simulink model "quad_waypoint_schedule"  (R2020a)
settings: Solver=FixedStepAuto  StartTime=0.0  StopTime=10.0  RelTol=1e-3
undefined symbols (not defined in the file): sim_freq, threshold, waypoints, waypoints_time
libraries: simulink x1
settings Model: Creator=francois  LastModifiedBy=murray

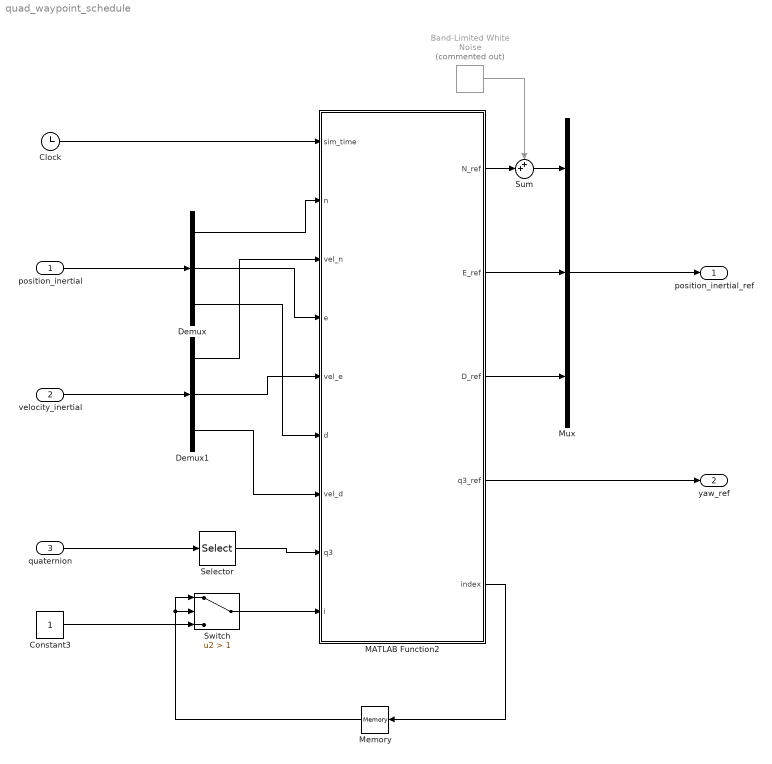
== system quad_waypoint_schedule ==
  position_inertial : Inport
  velocity_inertial : Inport  Port=2
  quaternion : Inport  Port=3
  Band-Limited White Noise : simulink/Sources/Band-Limited White Noise  Commented=on  Cov=1e-6  Ts=1/sim_freq  seed=[23341]
  Clock : Clock
  Constant3 : Constant
  Demux : Demux  Outputs=3
  Demux1 : Demux  Outputs=3
  MATLAB Function2 : MATLAB Function  TreatAsAtomicUnit=on  SystemSampleTime=1/sim_freq
  Memory : Memory
  Mux : Mux  Inputs=3
  Selector : Selector  InputPortWidth=4  IndexOptions=Index vector (dialog)  Indices=[4]  OutputSizes=1
  Sum : Sum  Inputs=++|
  Switch : Switch  Criteria=u2 > Threshold  Threshold=1  InputSameDT=on
  position_inertial_ref : Outport  VectorParamsAs1DForOutWhenUnconnected=off
  yaw_ref : Outport  Port=2  VectorParamsAs1DForOutWhenUnconnected=off
  wires:
  Demux/3 -> MATLAB Function2/6(d)
  Sum/1 -> Mux/1
  Demux1/3 -> MATLAB Function2/7(vel_d)
  quaternion/1 -> Selector/1
  Demux/1 -> MATLAB Function2/2(n)
  Clock/1 -> MATLAB Function2/1(sim_time)
  Demux1/2 -> MATLAB Function2/5(vel_e)
  MATLAB Function2/3(D_ref) -> Mux/3
  MATLAB Function2/5(index) -> Memory/1
  MATLAB Function2/2(E_ref) -> Mux/2
  Switch/1 -> MATLAB Function2/9(i)
  Memory/1 -> Switch/2, Switch/1
  Demux/2 -> MATLAB Function2/4(e)
  Mux/1 -> position_inertial_ref/1
  position_inertial/1 -> Demux/1
  Constant3/1 -> Switch/3
  Band-Limited White Noise/1 -> Sum/1
  Demux1/1 -> MATLAB Function2/3(vel_n)
  MATLAB Function2/1(N_ref) -> Sum/2
  Selector/1 -> MATLAB Function2/8(q3)
  MATLAB Function2/4(q3_ref) -> yaw_ref/1
  velocity_inertial/1 -> Demux1/1

== matlab function quad_waypoint_schedule/MATLAB Function2 ==
  data: sim_time input; n input; vel_n input; N_ref output; e input; vel_e input; d input; vel_d input; q3 input; i input; E_ref output; D_ref output; q3_ref output; index output; waypoints parameter; threshold parameter; waypoints_time parameter
function [N_ref, E_ref, D_ref, q3_ref, index] = waypoint_scheduler(sim_time, n, vel_n, e, vel_e, d, vel_d, q3, i, waypoints, threshold, waypoints_time)
    if i > 1
        index = floor(i); % ensure index is an positive integer
    else
        index = 1;
    end

    if waypoints_time(index) < 0
        if ((abs(waypoints(index, 1) - n) < threshold) && abs(vel_n) < threshold) && ((abs(waypoints(index, 2) - e) < threshold && abs(vel_e) < threshold)) && ((abs(waypoints(index, 3) - d) < threshold && abs(vel_d) < threshold))
            if index < length(waypoints(:,1))
                index = index + 1;
            end
        end
    else
        if mod(sim_time, waypoints_time(index)) == 0 % Only at intervals given by waypoint time. %%% Note 
            if index < length(waypoints(:,1))
                index = index + 1;
            end
        end
    end

    N_ref = waypoints(index, 1);
    E_ref = waypoints(index, 2);
    D_ref = waypoints(index, 3);
    q3_ref = 0;

end
